simulink model "OPENXWD"  (R2022b)
settings: Solver=VariableStepAuto  StartTime=0.0  StopTime=inf  RelTol=1e-3  EnableMultiTasking=on
PreLoadFcn:
  | run('Parameters\FSE_Parameters.m')
values from neighbouring files (symbols this model uses):
  batt_curr = 1    [srcipt.m]
  batt_voltage = 587    [srcipt.m]
  drive_ratio = 14.25    [srcipt.m]
  g = 9.81    [srcipt.m]
  h = 0.25    [srcipt.m]
  Ku = 1/500*-1    (= -0.002)    [srcipt.m]
  L = 1.53    [srcipt.m]
  lf = L-lr    (= 0.765)    [srcipt.m]
  lr = 0.765    [srcipt.m]
  ls = 1.242    [srcipt.m]
  m = 226    [srcipt.m]
  max_moment = 9.8    [srcipt.m]
  Mz_I = 70    [srcipt.m]
  Mz_p = 700    [srcipt.m]
  P_max = 80000    [srcipt.m]
  rw = 0.217    [srcipt.m]
libraries: CarMaker4SL x44, simulink x1
(part 3 of 3)

== system OPENXWD/CarMaker/IPG Vehicle/The Best TorqueVectoring/TorqueVectoring/Regenerative braking/Tmax ==
  Add : Sum  Inputs=++++
  Divide : Product  Inputs=*/
  Dot Product : DotProduct  OutDataTypeStr=Inherit: Inherit via internal rule
  Gain : Gain  Gain=0.95
  I_max : Constant  Value=15
  Read CM Dict : CarMaker4SL/Read CM Dict  xname=Car.WheelSpd_FR  xsync=off  xstime=Continuous
  Read CM Dict7 : CarMaker4SL/Read CM Dict  xname=Car.WheelSpd_FL  xsync=off  xstime=Continuous
  Read CM Dict8 : CarMaker4SL/Read CM Dict  xname=Car.WheelSpd_RL  xsync=off  xstime=Continuous
  Read CM Dict9 : CarMaker4SL/Read CM Dict  xname=Car.WheelSpd_RR  xsync=off  xstime=Continuous
  Vdc : Constant  Value=550
  Output : Outport
  wires:
  Dot Product/1 -> Gain/1
  Read CM Dict9/1 -> Add/4
  Read CM Dict7/1 -> Add/1
  Read CM Dict8/1 -> Add/3
  Read CM Dict/1 -> Add/2
  Add/1 -> Divide/2
  Vdc/1 -> Dot Product/2
  Divide/1 -> Output/1
  I_max/1 -> Dot Product/1
  Gain/1 -> Divide/1

== system OPENXWD/CarMaker/IPG Vehicle/The Best TorqueVectoring/TorqueVectoring/Torque distribution Tv/Fzfl ==
  ax : Inport
  ay : Inport  Port=2
  Constant : Constant  Value=g*lr
  Gain : Gain  Gain=m/(2*L)
  Gain1 : Gain  Gain=h
  Gain2 : Gain  Gain=(h*lr)/(ls)
  Sum : Sum  Inputs=+--
  Fzfl : Outport
  wires:
  Sum/1 -> Gain/1
  Constant/1 -> Sum/1
  Gain1/1 -> Sum/2
  ax/1 -> Gain1/1
  ay/1 -> Gain2/1
  Gain2/1 -> Sum/3
  Gain/1 -> Fzfl/1

== system OPENXWD/CarMaker/IPG Vehicle/The Best TorqueVectoring/TorqueVectoring/Torque distribution Tv/Fzfr ==
  ay : Inport
  ax : Inport  Port=2
  Constant : Constant  Value=g*lr
  Gain : Gain  Gain=m/(2*L)
  Gain1 : Gain  Gain=h
  Gain2 : Gain  Gain=(h*lr)/(ls)
  Sum : Sum  Inputs=+-+
  Fzfr : Outport
  wires:
  Sum/1 -> Gain/1
  Constant/1 -> Sum/1
  Gain1/1 -> Sum/2
  ax/1 -> Gain1/1
  ay/1 -> Gain2/1
  Gain2/1 -> Sum/3
  Gain/1 -> Fzfr/1

== system OPENXWD/CarMaker/IPG Vehicle/The Best TorqueVectoring/TorqueVectoring/Torque distribution Tv/Fzrl ==
  ax : Inport
  ay : Inport  Port=2
  Constant : Constant  Value=g*lf
  Gain : Gain  Gain=m/(2*L)
  Gain1 : Gain  Gain=h
  Gain2 : Gain  Gain=(h*lf)/(ls)
  Sum : Sum  Inputs=++-
  Fzrl : Outport
  wires:
  Gain/1 -> Fzrl/1
  Gain2/1 -> Sum/3
  ay/1 -> Gain2/1
  Sum/1 -> Gain/1
  Constant/1 -> Sum/1
  ax/1 -> Gain1/1
  Gain1/1 -> Sum/2

== system OPENXWD/CarMaker/IPG Vehicle/The Best TorqueVectoring/TorqueVectoring/Torque distribution Tv/Fzrr ==
  ay : Inport
  ax : Inport  Port=2
  Constant : Constant  Value=g*lf
  Gain : Gain  Gain=m/(2*L)
  Gain1 : Gain  Gain=h
  Gain2 : Gain  Gain=(h*lf)/(ls)
  Sum : Sum  Inputs=+++
  Fzrr : Outport
  wires:
  Gain/1 -> Fzrr/1
  Gain2/1 -> Sum/3
  ay/1 -> Gain2/1
  Sum/1 -> Gain/1
  Constant/1 -> Sum/1
  ax/1 -> Gain1/1
  Gain1/1 -> Sum/2

== system OPENXWD/CarMaker/IPG Vehicle/The Best TorqueVectoring/TorqueVectoring/Torque distribution Tv/T_FL ==
  Fzfl : Inport
  Tt : Inport  Port=2
  ^Mz : Inport  Port=3
  Gain : Gain  Gain=rw/ls
  Gain1 : Gain  Gain=1/(m*g)
  Product : Product
  Sum : Sum  Inputs=+-
  T_FL : Outport
  wires:
  Gain/1 -> Sum/2
  Tt/1 -> Sum/1
  ^Mz/1 -> Gain/1
  Fzfl/1 -> Gain1/1
  Gain1/1 -> Product/1
  Product/1 -> T_FL/1
  Sum/1 -> Product/2

== system OPENXWD/CarMaker/IPG Vehicle/The Best TorqueVectoring/TorqueVectoring/Torque distribution Tv/T_FR ==
  Fzfr : Inport
  Tt : Inport  Port=2
  ^Mz : Inport  Port=3
  Gain : Gain  Gain=rw/ls
  Gain1 : Gain  Gain=1/(m*g)
  Product : Product
  Sum : Sum
  T_FR : Outport
  wires:
  Gain/1 -> Sum/2
  Tt/1 -> Sum/1
  ^Mz/1 -> Gain/1
  Fzfr/1 -> Gain1/1
  Gain1/1 -> Product/1
  Product/1 -> T_FR/1
  Sum/1 -> Product/2

== system OPENXWD/CarMaker/IPG Vehicle/The Best TorqueVectoring/TorqueVectoring/Torque distribution Tv/T_FR1 ==
  FzRR : Inport
  Tt : Inport  Port=2
  ^Mz : Inport  Port=3
  Gain : Gain  Gain=rw/ls
  Gain1 : Gain  Gain=1/(m*g)
  Product : Product
  Sum : Sum
  T_RR : Outport
  wires:
  Gain/1 -> Sum/2
  Tt/1 -> Sum/1
  ^Mz/1 -> Gain/1
  FzRR/1 -> Gain1/1
  Gain1/1 -> Product/1
  Product/1 -> T_RR/1
  Sum/1 -> Product/2

== system OPENXWD/CarMaker/IPG Vehicle/The Best TorqueVectoring/TorqueVectoring/Torque distribution Tv/T_RL ==
  FzRL : Inport
  Tt : Inport  Port=2
  ^Mz : Inport  Port=3
  Gain : Gain  Gain=rw/ls
  Gain1 : Gain  Gain=1/(m*g)
  Product : Product
  Sum : Sum  Inputs=+-
  T_RL : Outport
  wires:
  Gain/1 -> Sum/2
  Tt/1 -> Sum/1
  ^Mz/1 -> Gain/1
  FzRL/1 -> Gain1/1
  Gain1/1 -> Product/1
  Product/1 -> T_RL/1
  Sum/1 -> Product/2
